simulink model "sim5_3"  (R2019a)
settings: Solver=VariableStepAuto  StartTime=0.0  StopTime=10.0  RelTol=1e-3
values from neighbouring files (symbols this model uses):
  C_2 = [1 0; 0 1]    [matlab_5_3.m]
  D_2 = [0; 0]    [matlab_5_3.m]
  den = [1 1 0]    [matlab_5_3.m]
  den_d = [1 -1.3679, 0.3679]    [matlab_5_3.m]
  h = 1    [matlab_5_3.m]
  K = 0.391    [matlab_5_3.m]
  num = [1]    [matlab_5_3.m]
  num_d = [0.3679, 0.2642]    [matlab_5_3.m]
undefined symbols (not defined in the file or in its folder): A, B, C, D, gama, phi
settings Model: Creator=User  LastModifiedBy=User

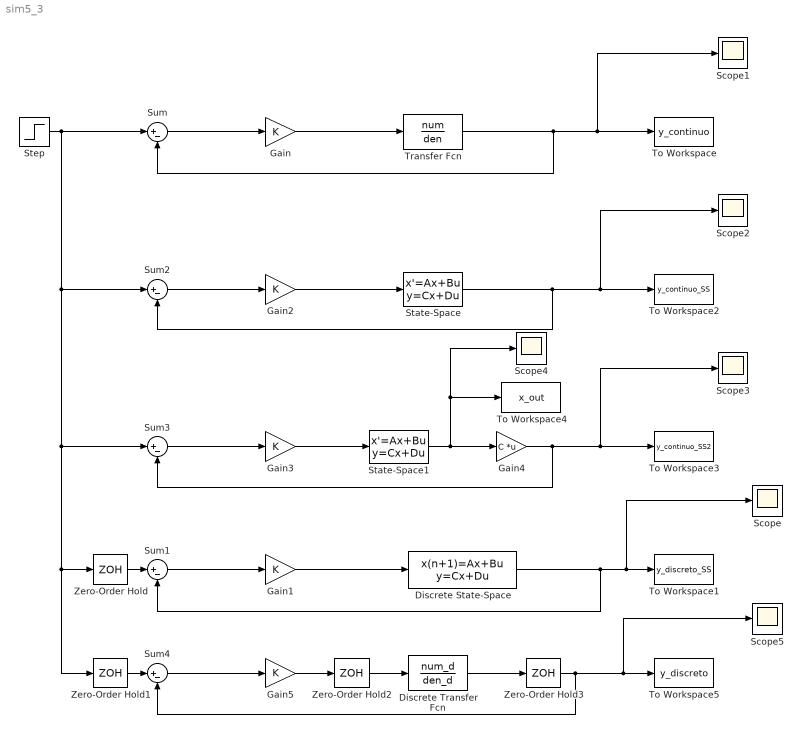
== system sim5_3 ==
  Discrete Transfer Fcn : DiscreteTransferFcn  Numerator=num_d  Denominator=den_d  SampleTime=h
  Discrete State-Space : DiscreteStateSpace  A=phi  B=gama  C=C  D=D  SampleTime=-1
  Gain{,1..3,5} (5 alike) : Gain  Gain=K
  Gain4 : Gain  Gain=C  Multiplication=Matrix(K*u)
  Scope{,1..5} (6 alike) : Scope
  State-Space : StateSpace  A=A  B=B  C=C  D=D  InitialCondition=0
  State-Space1 : StateSpace  A=A  B=B  C=C_2  D=D_2  InitialCondition=0
  Step : Step  Time=0  SampleTime=0
  Sum{,1..4} (5 alike) : Sum  Inputs=|+-
  To Workspace : ToWorkspace  VariableName=y_continuo  SaveFormat=Structure With Time  SampleTime=-1
  To Workspace1 : ToWorkspace  VariableName=y_discreto_SS  SaveFormat=Structure With Time  SampleTime=-1
  To Workspace2 : ToWorkspace  VariableName=y_continuo_SS  SaveFormat=Structure With Time  SampleTime=-1
  To Workspace3 : ToWorkspace  VariableName=y_continuo_SS2  SaveFormat=Structure With Time  SampleTime=-1
  To Workspace4 : ToWorkspace  VariableName=x_out  SaveFormat=Structure With Time  SampleTime=-1
  To Workspace5 : ToWorkspace  VariableName=y_discreto  SaveFormat=Structure With Time  SampleTime=-1
  Transfer Fcn : TransferFcn  Numerator=num  Denominator=den
  Zero-Order Hold : ZeroOrderHold  SampleTime=h
  Zero-Order Hold1 : ZeroOrderHold  SampleTime=-1
  Zero-Order Hold2 : ZeroOrderHold  SampleTime=-1
  Zero-Order Hold3 : ZeroOrderHold  SampleTime=-1
  wires:
  Transfer Fcn/1 -> Sum/2, Scope1/1, To Workspace/1
  Gain/1 -> Transfer Fcn/1
  Sum/1 -> Gain/1
  Step/1 -> Zero-Order Hold1/1, Zero-Order Hold/1, Sum3/1, Sum2/1, Sum/1
  Zero-Order Hold/1 -> Sum1/1
  Sum1/1 -> Gain1/1
  Discrete State-Space/1 -> Sum1/2, Scope/1, To Workspace1/1
  Gain2/1 -> State-Space/1
  Sum2/1 -> Gain2/1
  State-Space/1 -> Scope2/1, To Workspace2/1, Sum2/2
  Gain3/1 -> State-Space1/1
  Sum3/1 -> Gain3/1
  Gain4/1 -> Scope3/1, To Workspace3/1, Sum3/2
  State-Space1/1 -> To Workspace4/1, Scope4/1, Gain4/1
  Gain1/1 -> Discrete State-Space/1
  Zero-Order Hold1/1 -> Sum4/1
  Sum4/1 -> Gain5/1
  Gain5/1 -> Zero-Order Hold2/1
  Zero-Order Hold2/1 -> Discrete Transfer Fcn/1
  Discrete Transfer Fcn/1 -> Zero-Order Hold3/1
  Zero-Order Hold3/1 -> Sum4/2, Scope5/1, To Workspace5/1
